simulink model "Levitatore_NonLineare"  (R2013a)
settings: Solver=ode45  StartTime=0.0  StopTime=10.0  RelTol=1e-3
values from neighbouring files (symbols this model uses):
  g = 9.81*m/s^2    (= 9.81)    [prova.m]
  K_0 = 4*N*m^2    (= 4)    [prova.m]
  K_m = 5*N*(m^2)*Amp^-2    (= 5)    [prova.m]
  K_v = 1*V/m    (= 1)    [prova.m]
  M = 5*Kg    (= 5)    [prova.m]
  v_0 = 2*V    (= 2)    [prova.m]
settings Model: Creator=peppe  LastModifiedBy=peppe

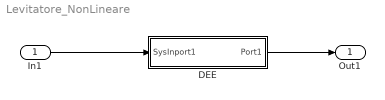
== system Levitatore_NonLineare ==
  In1 : Inport
  DEE : Subsystem  mask(Differential Equation Editor (DEE)){}
      settings: OpenFcn=diffeqed
      mask Display: disp('Differential Equation\n Editor')
  Out1 : Outport
  wires:
  In1/1 -> DEE/1(SysInport1)
  DEE/1(Port1) -> Out1/1

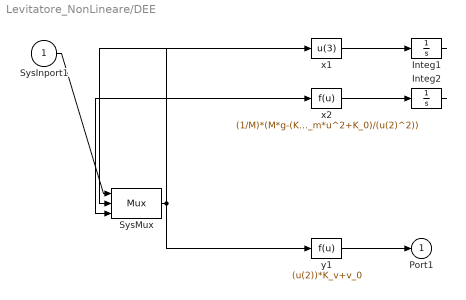
== system Levitatore_NonLineare/DEE ==
  SysInport1 : Inport
  Integ1 : Integrator
  Integ2 : Integrator
  SysMux : Mux  Inputs=3
  x1 : Fcn  Expr=u(3)
  x2 : Fcn  Expr=(1/M)*(M*g-(K_m*u^2+K_0)/(u(2)^2))
  y1 : Fcn  Expr=(u(2))*K_v+v_0
  Port1 : Outport
  wires:
  SysInport1/1 -> SysMux/1
  SysMux/1 -> x1/1, x2/1, y1/1
  x1/1 -> Integ1/1
  Integ1/1 -> SysMux/2
  x2/1 -> Integ2/1
  Integ2/1 -> SysMux/3
  y1/1 -> Port1/1
